simulink model "SimulationModel"  (R2019b)
settings: Solver=VariableStepAuto  StartTime=0.0  StopTime=10.0  RelTol=1e-3
PostLoadFcn:
  | helperCreateVehicleTrajectories
InitFcn:
  | helperCreateVehicleTrajectories
StopFcn:
  | initTrajectories=true;
libraries: sim3dprobsensorlib x7, sim3dautolib x6, drivinglib x2, sim3dlib x1
CloseFcn:
  | clear
settings Model: Creator=The MathWorks, Inc.  LastModifiedBy=Raymo
settings DebuggingCC: SymbolicDimsDataTypeCodeGenerationDiagnostic=none

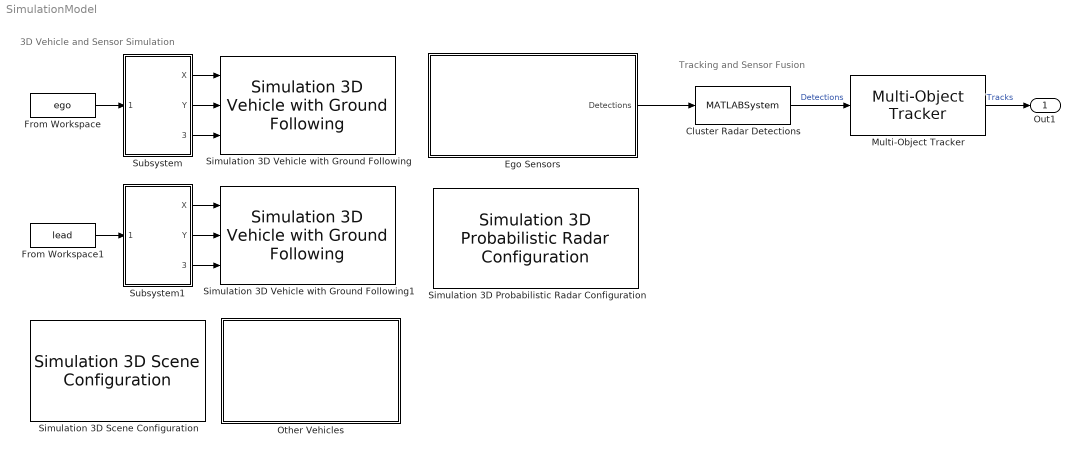
== system SimulationModel ==
  note: Tracking and Sensor Fusion
  note: 3D Vehicle and Sensor Simulation
  Cluster Radar Detections : MATLABSystem  System=helperClusterDetections  ClusterSize=5  BusNameSource=Auto  BusName=BusClusterDetections  SimulateUsing=Interpreted execution
      mask Type: helperClusterDetections
      mask Display:
      | disp(['Detection' char(10) 'Clustering']);
      | port_label('input',1,'In');
      | port_label('output',1,'Out');
  Ego Sensors : Subsystem
  From Workspace : FromWorkspace  VariableName=ego  OutDataTypeStr=Bus: BusActorPose  SampleTime=0.1
  From Workspace1 : FromWorkspace  VariableName=lead  OutDataTypeStr=Bus: BusActorPose  SampleTime=0.1
  Multi-Object Tracker : drivinglib/Multi-Object Tracker  FilterInitializationFcn=helperInitSimulinkDemoFilter  AssignmentThreshold=50  ConfirmationParameters=[ 2, 3 ]  NumCoastingUpdates=5  MaxNumTracks=20  MaxNumSensors=8  TimeInputSource=Auto  HasCostMatrixInput=off  BusNameSource=Property  BusName=BusMultiObjectTracker1  TentativeTracksOutputPort=off  AllTracksOutputPort=off  SimulateUsing=Interpreted execution
      settings: SourceProductName=Automated Driving Toolbox  SourceProductBaseCode=DR
  Other Vehicles : Subsystem
  Simulation 3D Probabilistic Radar Configuration : sim3dprobsensorlib/Simulation 3D Probabilistic Radar Configuration  RCSactorKeys=[10]  RCSactorProfiles={[10, 10;10, 10]}  RCSdefaultValue=-20  aMode=3
      settings: SourceProductName=Automated Driving Toolbox  SourceProductBaseCode=DR
  Simulation 3D Scene Configuration : sim3dlib/Simulation 3D Scene Configuration  SceneDesc=Curved road  vehTagList={'Scene Origin';'SimulinkVehicle1';'SimulinkVehicle2';'SimulinkVehicle3';'SimulinkVehicle4';'SimulinkVehicle5';'SimulinkVehicle6'}  vehTag=SimulinkVehicle1  OpVisEn=off  Ts=0.1  ProjectFormat=Executable  ProjectName=VehicleSimulation.exe  sensorTag=MainCamera1  sensorId=1  sensorName=MainCamera1  mountLoc=Origin  offsetFlag=off  tmountOffset=[0, 0, 0]  rmountOffset=[0, 0, 0]  HorizontalResolution=1280  VerticalResolution=720  HorizontalFOV=60  mountPoint=[0 0 0]  mountOrientation=[0 0 0]  aMode=3  ID=1
      settings: SourceProductName=Automated Driving Toolbox  SourceProductBaseCode=DR
  Simulation 3D Vehicle with Ground Following : sim3dautolib/Simulation 3D Vehicle with Ground Following  Priority=-1  PassVehMesh=Muscle car  VehColor=Yellow  InitialPos=[0, 0, 0]  InitialRot=[0, 0, 0]  ActorName=SimulinkVehicle1  SampleTime=-1  ActorType=SimulinkVehicle  ID=1  aMode=3  ActorTag=SimulinkVehicle1  CoordinateScheme=ISO  TransformOutportEnabled=off
      settings: SourceProductName=Automated Driving Toolbox  SourceProductBaseCode=DR
  Simulation 3D Vehicle with Ground Following1 : sim3dautolib/Simulation 3D Vehicle with Ground Following  Priority=-1  PassVehMesh=Sedan  VehColor=Silver  InitialPos=[0, 0, 0]  InitialRot=[0, 0, 0]  ActorName=SimulinkVehicle2  SampleTime=-1  ActorType=SimulinkVehicle  ID=2  aMode=3  ActorTag=SimulinkVehicle2  CoordinateScheme=ISO  TransformOutportEnabled=off
      settings: SourceProductName=Automated Driving Toolbox  SourceProductBaseCode=DR
  Subsystem : Subsystem
  Subsystem1 : Subsystem
  Out1 : Outport  VectorParamsAs1DForOutWhenUnconnected=off
  wires:
  Subsystem1/3(<Yaw>) -> Simulation 3D Vehicle with Ground Following1/3
  Subsystem/3(<Yaw>) -> Simulation 3D Vehicle with Ground Following/3
  Subsystem/2(Y) -> Simulation 3D Vehicle with Ground Following/2
  Cluster Radar Detections/1 -> Multi-Object Tracker/1  "Detections"
  Subsystem/1(X) -> Simulation 3D Vehicle with Ground Following/1
  Subsystem1/2(Y) -> Simulation 3D Vehicle with Ground Following1/2
  From Workspace1/1 -> Subsystem1/1(ActorPose)
  From Workspace/1 -> Subsystem/1(ActorPose)
  Multi-Object Tracker/1 -> Out1/1  "Tracks"
  Subsystem1/1(X) -> Simulation 3D Vehicle with Ground Following1/1
  Ego Sensors/1(Detections) -> Cluster Radar Detections/1

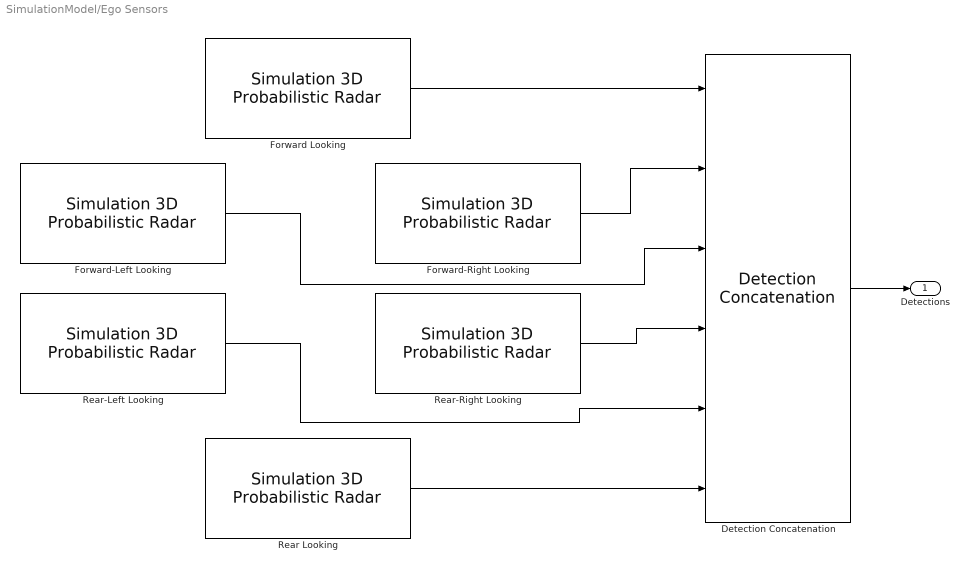
== system SimulationModel/Ego Sensors ==
  Detection Concatenation : drivinglib/Detection Concatenation  NumInputs=6  BusNameSource=Auto  BusName=BusDetectionConcatenation  SimulateUsing=Interpreted execution
      settings: SourceProductName=Automated Driving Toolbox  SourceProductBaseCode=DR
  Forward Looking : sim3dprobsensorlib/Simulation 3D Probabilistic Radar  Priority=1  sensorTag=Sim3dSensor1  sensorId=1  sensorName=Sim3dSensor1  vehTagList={'SimulinkVehicle1';'SimulinkVehicle2';'SimulinkVehicle3';'SimulinkVehicle4';'SimulinkVehicle5';'SimulinkVehicle6';'root'}  vehTag=SimulinkVehicle1  mountLoc=Front bumper  offsetFlag=off  tmountOffset=[0, 0, 0]  rmountOffset=[0, 0, 0]  AzimuthResolution=4  ElevationResolution=10  RangeResolution=2.5  RangeRateResolution=0.5  AzimuthBiasFraction=0.1  ElevationBiasFraction=0.1  RangeBiasFraction=0.05  RangeRateBiasFraction=0.05  FieldOfView=[ 45, 5 ]  DetectionRange=[ 1, 150 ]  RangeRateLimits=[ -100, 100 ]  DetectionProbability=0.9  FalseAlarmRate=1e-6  ReferenceRange=100  ReferenceRCS=0  HasElevation=off  HasRangeRate=on  HasNoise=on  HasFalseAlarms=on  InitialSeedSource=Repeatable  InitialSeed=0  MaxNumDetections=50  DetectionCoordinates=Ego Cartesian  SpecifyOutputBusName=off  BusName=BusSimulation3DRadarTruthSensor  SampleTime=0.1  mountPoint=[2.47350001335144 0 0.439999997615814]  mountOrientation=[0 0 0]  aMode=3  ID=1
      settings: SourceProductName=Automated Driving Toolbox  SourceProductBaseCode=DR
  Forward-Left Looking : sim3dprobsensorlib/Simulation 3D Probabilistic Radar  Priority=1  sensorTag=Sim3dSensor5  sensorId=5  sensorName=Sim3dSensor5  vehTagList={'Scene Origin';'SimulinkVehicle1';'SimulinkVehicle2';'SimulinkVehicle3';'SimulinkVehicle4';'SimulinkVehicle5';'SimulinkVehicle6'}  vehTag=SimulinkVehicle1  mountLoc=Front bumper  offsetFlag=on  tmountOffset=[0, 0.9, 0]  rmountOffset=[0, 0, 60]  AzimuthResolution=4  ElevationResolution=10  RangeResolution=2.5  RangeRateResolution=0.5  AzimuthBiasFraction=0.1  ElevationBiasFraction=0.1  RangeBiasFraction=0.05  RangeRateBiasFraction=0.05  FieldOfView=[ 90, 5 ]  DetectionRange=[ 1, 30 ]  RangeRateLimits=[ -100, 100 ]  DetectionProbability=0.9  FalseAlarmRate=1e-6  ReferenceRange=100  ReferenceRCS=0  HasElevation=off  HasRangeRate=on  HasNoise=on  HasFalseAlarms=on  InitialSeedSource=Repeatable  InitialSeed=0  MaxNumDetections=50  DetectionCoordinates=Ego Cartesian  SpecifyOutputBusName=off  BusName=BusSimulation3DRadarTruthSensor  SampleTime=0.1  mountPoint=[2.47350001335144 -0.899999976158142 0.439999997615814]  mountOrientation=[0 0 -60]  aMode=3  ID=5
      settings: SourceProductName=Automated Driving Toolbox  SourceProductBaseCode=DR
  Forward-Right Looking : sim3dprobsensorlib/Simulation 3D Probabilistic Radar  Priority=1  sensorTag=Sim3dSensor6  sensorId=6  sensorName=Sim3dSensor6  vehTagList={'Scene Origin';'SimulinkVehicle1';'SimulinkVehicle2'}  vehTag=SimulinkVehicle1  mountLoc=Front bumper  offsetFlag=on  tmountOffset=[0, -0.9, 0]  rmountOffset=[0, 0, -60]  AzimuthResolution=4  ElevationResolution=10  RangeResolution=2.5  RangeRateResolution=0.5  AzimuthBiasFraction=0.1  ElevationBiasFraction=0.1  RangeBiasFraction=0.05  RangeRateBiasFraction=0.05  FieldOfView=[ 90, 5 ]  DetectionRange=[ 1, 30 ]  RangeRateLimits=[ -100, 100 ]  DetectionProbability=0.9  FalseAlarmRate=1e-6  ReferenceRange=100  ReferenceRCS=0  HasElevation=off  HasRangeRate=on  HasNoise=on  HasFalseAlarms=on  InitialSeedSource=Repeatable  InitialSeed=0  MaxNumDetections=50  DetectionCoordinates=Ego Cartesian  SpecifyOutputBusName=off  BusName=BusSimulation3DRadarTruthSensor  SampleTime=0.1  mountPoint=[2.47350001335144 0.899999976158142 0.439999997615814]  mountOrientation=[0 0 60]  aMode=3  ID=6
      settings: SourceProductName=Automated Driving Toolbox  SourceProductBaseCode=DR
  Rear Looking : sim3dprobsensorlib/Simulation 3D Probabilistic Radar  Priority=1  sensorTag=Sim3dSensor2  sensorId=2  sensorName=Sim3dSensor2  vehTagList={'SimulinkVehicle1';'SimulinkVehicle2';'root'}  vehTag=SimulinkVehicle1  mountLoc=Rear bumper  offsetFlag=off  tmountOffset=[0, 0, 0]  rmountOffset=[0, 0, 0]  AzimuthResolution=4  ElevationResolution=10  RangeResolution=2.5  RangeRateResolution=0.5  AzimuthBiasFraction=0.1  ElevationBiasFraction=0.1  RangeBiasFraction=0.05  RangeRateBiasFraction=0.05  FieldOfView=[ 45, 5 ]  DetectionRange=[ 1, 150 ]  RangeRateLimits=[ -100, 100 ]  DetectionProbability=0.9  FalseAlarmRate=1e-6  ReferenceRange=100  ReferenceRCS=0  HasElevation=off  HasRangeRate=on  HasNoise=on  HasFalseAlarms=on  InitialSeedSource=Repeatable  InitialSeed=0  MaxNumDetections=50  DetectionCoordinates=Ego Cartesian  SpecifyOutputBusName=off  BusName=BusSimulation3DRadarTruthSensor  SampleTime=0.1  mountPoint=[-2.47350001335144 0 0.439999997615814]  mountOrientation=[0 0 180]  aMode=3  ID=2
      settings: SourceProductName=Automated Driving Toolbox  SourceProductBaseCode=DR
  Rear-Left Looking : sim3dprobsensorlib/Simulation 3D Probabilistic Radar  Priority=1  sensorTag=Sim3dSensor3  sensorId=3  sensorName=Sim3dSensor3  vehTagList={'Scene Origin';'SimulinkVehicle1';'SimulinkVehicle2'}  vehTag=SimulinkVehicle1  mountLoc=Rear bumper  offsetFlag=on  tmountOffset=[0, 0.9, 0]  rmountOffset=[0, 0, -60]  AzimuthResolution=4  ElevationResolution=10  RangeResolution=2.5  RangeRateResolution=0.5  AzimuthBiasFraction=0.1  ElevationBiasFraction=0.1  RangeBiasFraction=0.05  RangeRateBiasFraction=0.05  FieldOfView=[ 90, 5 ]  DetectionRange=[ 1, 30 ]  RangeRateLimits=[ -100, 100 ]  DetectionProbability=0.9  FalseAlarmRate=1e-6  ReferenceRange=100  ReferenceRCS=0  HasElevation=off  HasRangeRate=on  HasNoise=on  HasFalseAlarms=on  InitialSeedSource=Repeatable  InitialSeed=0  MaxNumDetections=50  DetectionCoordinates=Ego Cartesian  SpecifyOutputBusName=off  BusName=BusSimulation3DRadarTruthSensor  SampleTime=0.1  mountPoint=[-2.47350001335144 -0.899999976158142 0.439999997615814]  mountOrientation=[0 0 240]  aMode=3  ID=3
      settings: SourceProductName=Automated Driving Toolbox  SourceProductBaseCode=DR
  Rear-Right Looking : sim3dprobsensorlib/Simulation 3D Probabilistic Radar  Priority=1  sensorTag=Sim3dSensor4  sensorId=4  sensorName=Sim3dSensor4  vehTagList={'Scene Origin';'SimulinkVehicle1';'SimulinkVehicle2'}  vehTag=SimulinkVehicle1  mountLoc=Rear bumper  offsetFlag=on  tmountOffset=[0, -0.9, 0]  rmountOffset=[0, 0, 60]  AzimuthResolution=4  ElevationResolution=10  RangeResolution=2.5  RangeRateResolution=0.5  AzimuthBiasFraction=0.1  ElevationBiasFraction=0.1  RangeBiasFraction=0.05  RangeRateBiasFraction=0.05  FieldOfView=[ 90, 5 ]  DetectionRange=[ 1, 30 ]  RangeRateLimits=[ -100, 100 ]  DetectionProbability=0.9  FalseAlarmRate=1e-6  ReferenceRange=100  ReferenceRCS=0  HasElevation=off  HasRangeRate=on  HasNoise=on  HasFalseAlarms=on  InitialSeedSource=Repeatable  InitialSeed=0  MaxNumDetections=50  DetectionCoordinates=Ego Cartesian  SpecifyOutputBusName=off  BusName=BusSimulation3DRadarTruthSensor  SampleTime=0.1  mountPoint=[-2.47350001335144 0.899999976158142 0.439999997615814]  mountOrientation=[0 0 120]  aMode=3  ID=4
      settings: SourceProductName=Automated Driving Toolbox  SourceProductBaseCode=DR
  Detections : Outport  VectorParamsAs1DForOutWhenUnconnected=off
  wires:
  Forward-Right Looking/1 -> Detection Concatenation/2
  Forward-Left Looking/1 -> Detection Concatenation/3
  Rear-Left Looking/1 -> Detection Concatenation/5
  Detection Concatenation/1 -> Detections/1
  Rear Looking/1 -> Detection Concatenation/6
  Rear-Right Looking/1 -> Detection Concatenation/4
  Forward Looking/1 -> Detection Concatenation/1

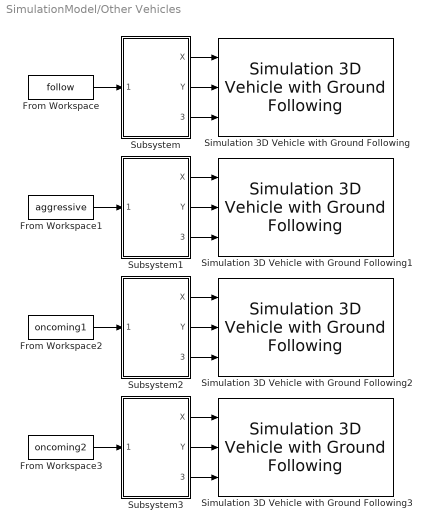
== system SimulationModel/Other Vehicles ==
  From Workspace : FromWorkspace  VariableName=follow  OutDataTypeStr=Bus: BusActorPose  SampleTime=0.1
  From Workspace1 : FromWorkspace  VariableName=aggressive  OutDataTypeStr=Bus: BusActorPose  SampleTime=0.1
  From Workspace2 : FromWorkspace  VariableName=oncoming1  OutDataTypeStr=Bus: BusActorPose  SampleTime=0.1
  From Workspace3 : FromWorkspace  VariableName=oncoming2  OutDataTypeStr=Bus: BusActorPose  SampleTime=0.1
  Simulation 3D Vehicle with Ground Following : sim3dautolib/Simulation 3D Vehicle with Ground Following  PassVehMesh=Sport utility vehicle  VehColor=Red  InitialPos=[0, 0, 0]  InitialRot=[0, 0, 0]  ActorName=SimulinkVehicle3  SampleTime=-1  ActorType=SimulinkVehicle  ID=3  aMode=3  ActorTag=SimulinkVehicle3  CoordinateScheme=ISO  TransformOutportEnabled=off
      settings: SourceProductName=Automated Driving Toolbox  SourceProductBaseCode=DR
  Simulation 3D Vehicle with Ground Following1 : sim3dautolib/Simulation 3D Vehicle with Ground Following  PassVehMesh=Small pickup truck  VehColor=Black  InitialPos=[0, 0, 0]  InitialRot=[0, 0, 0]  ActorName=SimulinkVehicle4  SampleTime=-1  ActorType=SimulinkVehicle  ID=4  aMode=3  ActorTag=SimulinkVehicle4  CoordinateScheme=ISO  TransformOutportEnabled=off
      settings: SourceProductName=Automated Driving Toolbox  SourceProductBaseCode=DR
  Simulation 3D Vehicle with Ground Following2 : sim3dautolib/Simulation 3D Vehicle with Ground Following  PassVehMesh=Sport utility vehicle  VehColor=Green  InitialPos=[0, 0, 0]  InitialRot=[0, 0, 0]  ActorName=SimulinkVehicle5  SampleTime=-1  ActorType=SimulinkVehicle  ID=5  aMode=3  ActorTag=SimulinkVehicle5  CoordinateScheme=ISO  TransformOutportEnabled=off
      settings: SourceProductName=Automated Driving Toolbox  SourceProductBaseCode=DR
  Simulation 3D Vehicle with Ground Following3 : sim3dautolib/Simulation 3D Vehicle with Ground Following  PassVehMesh=Hatchback  VehColor=Orange  InitialPos=[0, 0, 0]  InitialRot=[0, 0, 0]  ActorName=SimulinkVehicle6  SampleTime=-1  ActorType=SimulinkVehicle  ID=6  aMode=3  ActorTag=SimulinkVehicle6  CoordinateScheme=ISO  TransformOutportEnabled=off
      settings: SourceProductName=Automated Driving Toolbox  SourceProductBaseCode=DR
  Subsystem : Subsystem
  Subsystem1 : Subsystem
  Subsystem2 : Subsystem
  Subsystem3 : Subsystem
  wires:
  Subsystem/3(<Yaw>) -> Simulation 3D Vehicle with Ground Following/3
  Subsystem/1(X) -> Simulation 3D Vehicle with Ground Following/1
  Subsystem/2(Y) -> Simulation 3D Vehicle with Ground Following/2
  From Workspace/1 -> Subsystem/1(ActorPose)
  From Workspace1/1 -> Subsystem1/1(ActorPose)
  Subsystem1/2(Y) -> Simulation 3D Vehicle with Ground Following1/2
  Subsystem1/1(X) -> Simulation 3D Vehicle with Ground Following1/1
  Subsystem1/3(<Yaw>) -> Simulation 3D Vehicle with Ground Following1/3
  Subsystem2/3(<Yaw>) -> Simulation 3D Vehicle with Ground Following2/3
  Subsystem2/2(Y) -> Simulation 3D Vehicle with Ground Following2/2
  From Workspace2/1 -> Subsystem2/1(ActorPose)
  Subsystem2/1(X) -> Simulation 3D Vehicle with Ground Following2/1
  From Workspace3/1 -> Subsystem3/1(ActorPose)
  Subsystem3/2(Y) -> Simulation 3D Vehicle with Ground Following3/2
  Subsystem3/3(<Yaw>) -> Simulation 3D Vehicle with Ground Following3/3
  Subsystem3/1(X) -> Simulation 3D Vehicle with Ground Following3/1

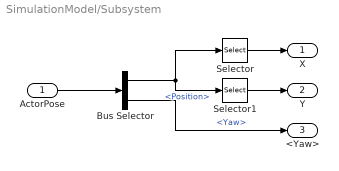
== system SimulationModel/Subsystem ==
  ActorPose : Inport
  Bus Selector : BusSelector  OutputSignals=Position,Yaw
  Selector : Selector  InputPortWidth=3  IndexOptions=Index vector (dialog)  Indices=1  OutputSizes=1
  Selector1 : Selector  InputPortWidth=3  IndexOptions=Index vector (dialog)  Indices=2  OutputSizes=1
  X : Outport  VectorParamsAs1DForOutWhenUnconnected=off
  Y : Outport  Port=2  VectorParamsAs1DForOutWhenUnconnected=off
  <Yaw> : Outport  Port=3  VectorParamsAs1DForOutWhenUnconnected=off
  wires:
  Bus Selector/1 -> Selector1/1, Selector/1  "<Position>"
  Bus Selector/2 -> <Yaw>/1  "<Yaw>"
  Selector/1 -> X/1
  Selector1/1 -> Y/1
  ActorPose/1 -> Bus Selector/1

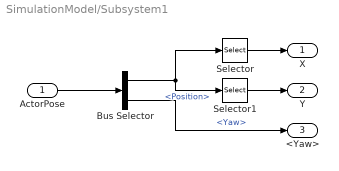
== system SimulationModel/Subsystem1 ==
  ActorPose : Inport
  Bus Selector : BusSelector  OutputSignals=Position,Yaw
  Selector : Selector  InputPortWidth=3  IndexOptions=Index vector (dialog)  Indices=1  OutputSizes=1
  Selector1 : Selector  InputPortWidth=3  IndexOptions=Index vector (dialog)  Indices=2  OutputSizes=1
  X : Outport  VectorParamsAs1DForOutWhenUnconnected=off
  Y : Outport  Port=2  VectorParamsAs1DForOutWhenUnconnected=off
  <Yaw> : Outport  Port=3  VectorParamsAs1DForOutWhenUnconnected=off
  wires:
  Bus Selector/1 -> Selector1/1, Selector/1  "<Position>"
  Bus Selector/2 -> <Yaw>/1  "<Yaw>"
  Selector/1 -> X/1
  Selector1/1 -> Y/1
  ActorPose/1 -> Bus Selector/1

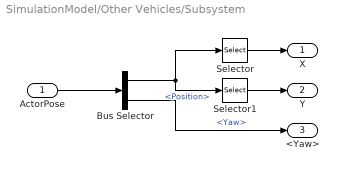
== system SimulationModel/Other Vehicles/Subsystem ==
  ActorPose : Inport
  Bus Selector : BusSelector  OutputSignals=Position,Yaw
  Selector : Selector  InputPortWidth=3  IndexOptions=Index vector (dialog)  Indices=1  OutputSizes=1
  Selector1 : Selector  InputPortWidth=3  IndexOptions=Index vector (dialog)  Indices=2  OutputSizes=1
  X : Outport  VectorParamsAs1DForOutWhenUnconnected=off
  Y : Outport  Port=2  VectorParamsAs1DForOutWhenUnconnected=off
  <Yaw> : Outport  Port=3  VectorParamsAs1DForOutWhenUnconnected=off
  wires:
  Bus Selector/1 -> Selector1/1, Selector/1  "<Position>"
  Bus Selector/2 -> <Yaw>/1  "<Yaw>"
  Selector/1 -> X/1
  Selector1/1 -> Y/1
  ActorPose/1 -> Bus Selector/1

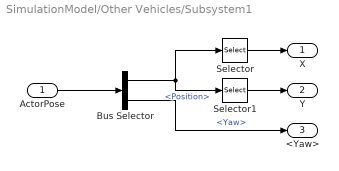
== system SimulationModel/Other Vehicles/Subsystem1 ==
  ActorPose : Inport
  Bus Selector : BusSelector  OutputSignals=Position,Yaw
  Selector : Selector  InputPortWidth=3  IndexOptions=Index vector (dialog)  Indices=1  OutputSizes=1
  Selector1 : Selector  InputPortWidth=3  IndexOptions=Index vector (dialog)  Indices=2  OutputSizes=1
  X : Outport  VectorParamsAs1DForOutWhenUnconnected=off
  Y : Outport  Port=2  VectorParamsAs1DForOutWhenUnconnected=off
  <Yaw> : Outport  Port=3  VectorParamsAs1DForOutWhenUnconnected=off
  wires:
  Bus Selector/1 -> Selector1/1, Selector/1  "<Position>"
  Bus Selector/2 -> <Yaw>/1  "<Yaw>"
  Selector/1 -> X/1
  Selector1/1 -> Y/1
  ActorPose/1 -> Bus Selector/1

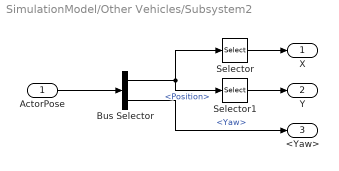
== system SimulationModel/Other Vehicles/Subsystem2 ==
  ActorPose : Inport
  Bus Selector : BusSelector  OutputSignals=Position,Yaw
  Selector : Selector  InputPortWidth=3  IndexOptions=Index vector (dialog)  Indices=1  OutputSizes=1
  Selector1 : Selector  InputPortWidth=3  IndexOptions=Index vector (dialog)  Indices=2  OutputSizes=1
  X : Outport  VectorParamsAs1DForOutWhenUnconnected=off
  Y : Outport  Port=2  VectorParamsAs1DForOutWhenUnconnected=off
  <Yaw> : Outport  Port=3  VectorParamsAs1DForOutWhenUnconnected=off
  wires:
  Bus Selector/1 -> Selector1/1, Selector/1  "<Position>"
  Bus Selector/2 -> <Yaw>/1  "<Yaw>"
  Selector/1 -> X/1
  Selector1/1 -> Y/1
  ActorPose/1 -> Bus Selector/1

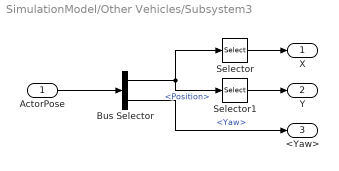
== system SimulationModel/Other Vehicles/Subsystem3 ==
  ActorPose : Inport
  Bus Selector : BusSelector  OutputSignals=Position,Yaw
  Selector : Selector  InputPortWidth=3  IndexOptions=Index vector (dialog)  Indices=1  OutputSizes=1
  Selector1 : Selector  InputPortWidth=3  IndexOptions=Index vector (dialog)  Indices=2  OutputSizes=1
  X : Outport  VectorParamsAs1DForOutWhenUnconnected=off
  Y : Outport  Port=2  VectorParamsAs1DForOutWhenUnconnected=off
  <Yaw> : Outport  Port=3  VectorParamsAs1DForOutWhenUnconnected=off
  wires:
  Bus Selector/1 -> Selector1/1, Selector/1  "<Position>"
  Bus Selector/2 -> <Yaw>/1  "<Yaw>"
  Selector/1 -> X/1
  Selector1/1 -> Y/1
  ActorPose/1 -> Bus Selector/1
